simulink model "general_Test_01"  (R2022b)
settings: Solver=VariableStepAuto  StartTime=0.0  StopTime=300.0  RelTol=1e-3
settings Model: Creator=umber  LastModifiedBy=umber
settings DataIOCC: ExternalInput=a.getElement('current')
settings ModelReferenceCC: EnableRefExpFcnMdlSchedulingChecks=on

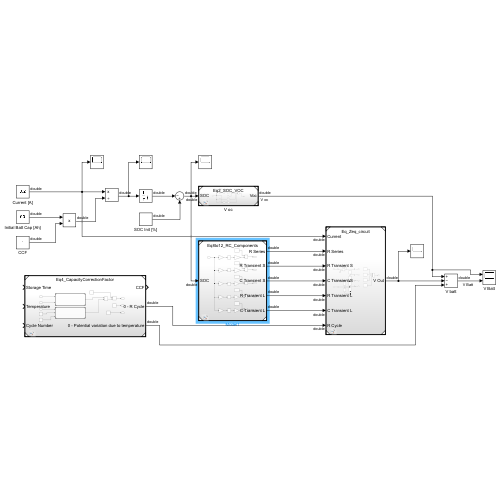
[thumbnail: Simulink's stored preview of the top-level diagram]
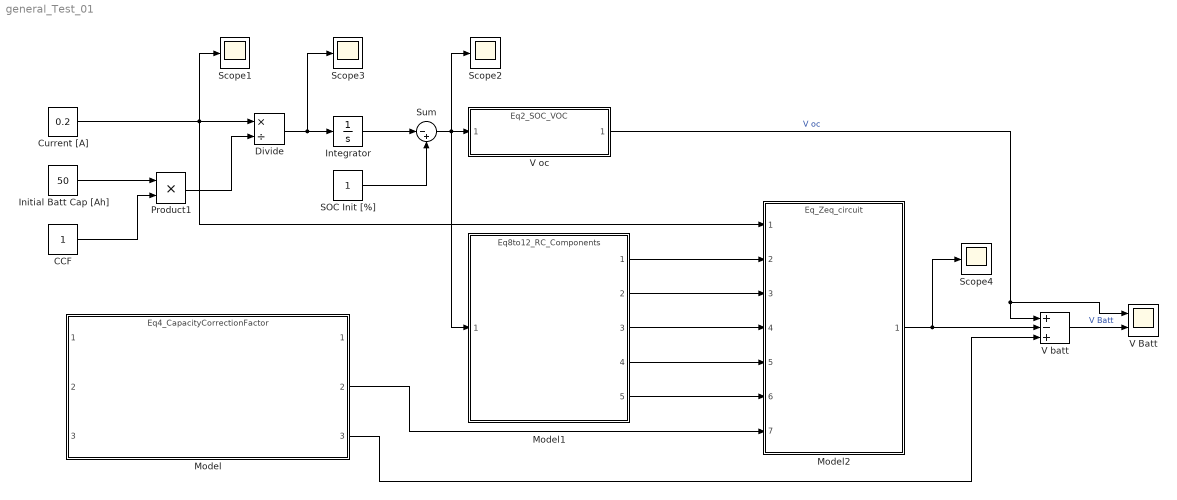
== system general_Test_01 ==
  CCF : Constant
  Current [A] : Constant  Value=0.2
  Divide : Product  Inputs=*/
  Initial Batt Cap [Ah] : Constant  Value=50
  Integrator : Integrator  LimitOutput=on  UpperSaturationLimit=1  LowerSaturationLimit=-1
  Model : ModelReference  ModelNameDialog=Eq4_CapacityCorrectionFactor.slx  SimulationMode=Normal  ModelReferenceVersion=2.0
  Model1 : ModelReference  ModelNameDialog=Eq8to12_RC_Components  SimulationMode=Normal  ModelReferenceVersion=2.0
  Model2 : ModelReference  ModelNameDialog=Eq_Zeq_circuit.slx  SimulationMode=Normal  ModelReferenceVersion=1.7
  Product1 : Product
  SOC Init [%] : Constant
  Scope{1..4} (4 alike) : Scope
  Sum : Sum  Inputs=|-+
  V Batt : Scope  NumInputPorts=2
  V batt : Sum  Inputs=+-+
  V oc : ModelReference  ModelNameDialog=Eq2_SOC_VOC.slx  SimulationMode=Normal  ModelReferenceVersion=1.3
  wires:
  Divide/1 -> Scope3/1, Integrator/1
  Integrator/1 -> Sum/1
  Sum/1 -> Scope2/1, Model1/1, V oc/1
  Current [A]/1 -> Scope1/1, Model2/1, Divide/1
  SOC Init [%]/1 -> Sum/2
  V oc/1 -> V Batt/1, V batt/1  "V oc"
  Model1/1 -> Model2/2
  Model/3 -> V batt/3
  Product1/1 -> Divide/2
  Initial Batt Cap [Ah]/1 -> Product1/1
  CCF/1 -> Product1/2
  Model2/1 -> Scope4/1, V batt/2
  Model1/2 -> Model2/3
  Model1/3 -> Model2/4
  Model1/4 -> Model2/5
  Model1/5 -> Model2/6
  Model/2 -> Model2/7
  V batt/1 -> V Batt/2  "V Batt"
